simulink model "Part1"  (R2016b)
settings: Solver=VariableStepAuto  StartTime=0.0  StopTime=10  FixedStep=.001  MaxStep=.1  RelTol=1e-3
settings Model: Creator=imi  LastModifiedBy=imi

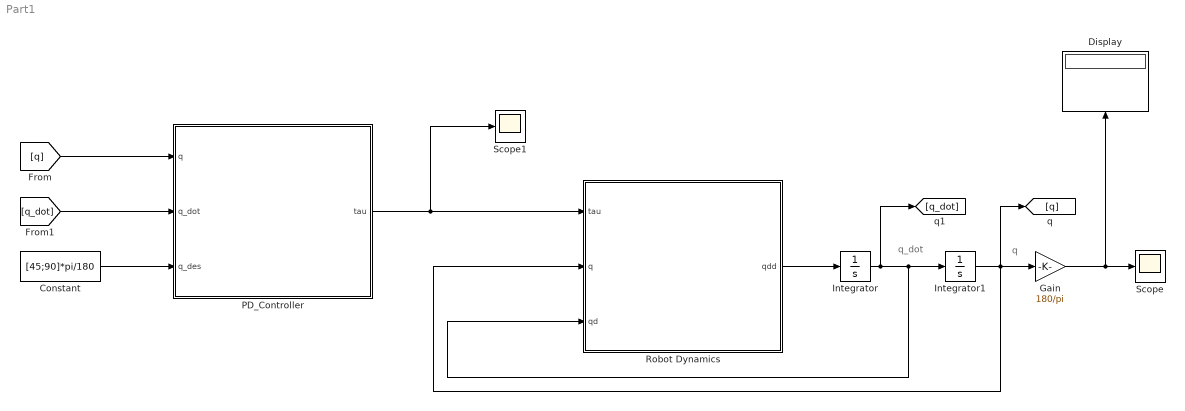
== system Part1 ==
  note: q
  note: q_dot
  Constant : Constant  Value=[45;90]*pi/180
  Display : Display
  Gain : Gain  Gain=180/pi
  Integrator : Integrator  InitialCondition=zeros(2,1)
  Integrator1 : Integrator  InitialCondition=[45;95]*pi/180*0
  PD_Controller : MATLAB Function  TreatAsAtomicUnit=on
  Robot Dynamics : MATLAB Function  TreatAsAtomicUnit=on
  Scope : Scope
  Scope1 : Scope
  wires:
  Integrator/1 -> [q_dot], Robot Dynamics/3(qd), Integrator1/1
  Robot Dynamics/1(qdd) -> Integrator/1
  Integrator1/1 -> [q], Gain/1, Robot Dynamics/2(q)
  PD_Controller/1(tau) -> Scope1/1, Robot Dynamics/1(tau)
  Gain/1 -> Scope/1, Display/1
  Constant/1 -> PD_Controller/3(q_des)
  [q] -> PD_Controller/1(q)
  [q_dot] -> PD_Controller/2(q_dot)

== matlab function Part1/PD_Controller ==
  data: q input; q_dot input; tau output; q_des input
function tau = fcn(q,q_dot,q_des)

Kp=20*eye(2);
Kd=2*eye(2);



tau=-Kp*(q-q_des)-Kd*q_dot;

== matlab function Part1/Robot Dynamics ==
  data: tau input; q input; qdd output; qd input
function qdd = fcn(tau,q,qd)

q1=q(1);
q2=q(2);

q1d=qd(1);
q2d=qd(2);



m1=.1;
m2=.1;

I1=.1;
I2=.1;

l1=.25;
l2=.12;

lc1=l1/2;
lc2=l2/2;


g=9.81;



d11=m1*lc1^2+m2*(l1^2+lc2^2+2*l1*lc2^2+2*l1*l2*cos(q2))+I1+I2;
d12=m2*(lc2^2+l1*l2*cos(q2))+I2;
d22=m2*lc2^2+I2;

h=-m2*l1*lc2*sin(q2);

c121=h;
c211=h;
c112=-h;
c221=h;



M=[d11,d12;d12,d22];
C=[c121*q2d,c211*q1d+c221*q2d;c112*q1d,0];
G=[(m1*lc1+m2*l1)*g*cos(q1)+m2*lc2*g*cos(q1+q2);m2*lc2*cos(q1+q2)];


qdd=pinv(M)*(tau-C*qd-G);
